simulink model "suspensionpassivetyredamper"  (R2016a)
settings: Solver=VariableStepAuto  StartTime=0.0  StopTime=10.0  RelTol=1e-3
undefined symbols (not defined in the file): b1, b2, k1, k2, m1, m2
settings Model: Creator=mm395  LastModifiedBy=mm395

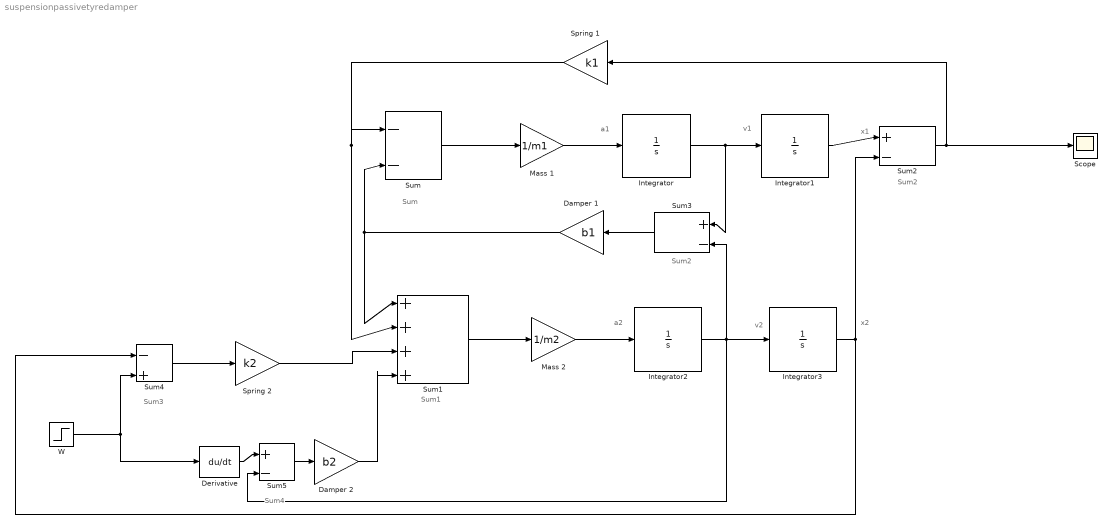
== system suspensionpassivetyredamper ==
  note: Sum3
  note: Sum1
  note: Sum
  note: x1
  note: v1
  note: a1
  note: x2
  note: v2
  note: a2
  note: Sum2
  note: Sum2
  note: Sum4
  Damper 1 : Gain  Gain=b1
  Damper 2 : Gain  Gain=b2
  Derivative : Derivative
  Integrator{,1..3} (4 alike) : Integrator
  Mass 1 : Gain  Gain=1/m1
  Mass 2 : Gain  Gain=1/m2
  Scope : Scope
  Spring 1 : Gain  Gain=k1
  Spring 2 : Gain  Gain=k2
  Sum : Sum  Inputs=|--
  Sum1 : Sum  Inputs=|++++
  Sum2 : Sum  Inputs=|+-
  Sum3 : Sum  Inputs=|+-
  Sum4 : Sum  Inputs=|-+
  Sum5 : Sum  Inputs=|+-
  W : Step  SampleTime=0
  wires:
  Mass 1/1 -> Integrator/1
  Integrator/1 -> Sum3/1, Integrator1/1
  Integrator1/1 -> Sum2/1
  Integrator3/1 -> Sum4/1, Sum2/2
  Sum/1 -> Mass 1/1
  Sum1/1 -> Mass 2/1
  Sum2/1 -> Scope/1, Spring 1/1
  Spring 1/1 -> Sum1/2, Sum/1
  Mass 2/1 -> Integrator2/1
  Integrator2/1 -> Sum5/2, Sum3/2, Integrator3/1
  Sum3/1 -> Damper 1/1
  Damper 1/1 -> Sum/2, Sum1/1
  Sum4/1 -> Spring 2/1
  Spring 2/1 -> Sum1/3
  W/1 -> Derivative/1, Sum4/2
  Derivative/1 -> Sum5/1
  Sum5/1 -> Damper 2/1
  Damper 2/1 -> Sum1/4
